simulink subsystem "Tank"  (R2019b)
settings: Solver=VariableStepAuto  StartTime=0.0  StopTime=10.0  RelTol=1e-3
settings Model: Creator=ovi  LastModifiedBy=ovi

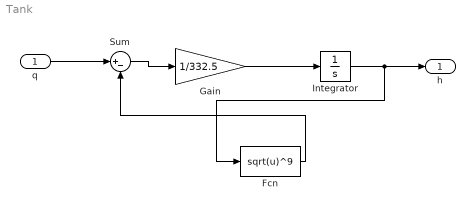
== system Tank ==
  q : Inport
  Fcn : Fcn  Expr=sqrt(u)^9
  Gain : Gain  Gain=1/332.5
  Integrator : Integrator
  Sum : Sum  Inputs=|+-
  h : Outport
  wires:
  q/1 -> Sum/1
  Sum/1 -> Gain/1
  Gain/1 -> Integrator/1
  Integrator/1 -> Fcn/1, h/1
  Fcn/1 -> Sum/2
